simulink model "automata_learning"  (R2022a)
settings: Solver=FixedStepAuto  StartTime=0.0  StopTime=10.0  FixedStep=0.005  RelTol=1e-3
settings Model: Creator=diego  LastModifiedBy=diego

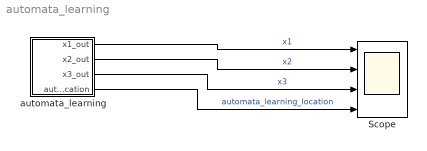
== system automata_learning ==
  Scope : Scope  NumInputPorts=4
  automata_learning : Stateflow chart  TreatAsAtomicUnit=on
  wires:
  automata_learning/1(x1_out) -> Scope/1  "x1"
  automata_learning/2(x2_out) -> Scope/2  "x2"
  automata_learning/3(x3_out) -> Scope/3  "x3"
  automata_learning/4(automata_learning_location) -> Scope/4  "automata_learning_location"

== stateflow chart automata_learning/automata_learning ==
  settings: updateMethod=CONTINUOUS
  state loc1
    du:
    x1_dot = 1801508832791591.0 * x1 * x2 / 9007199254740992.0 - 8444245416915159.0 * x2 / 1125899906842624.0 - 6192709348131975.0 * x3 / 1180591620717411300000.0 - 153051922812249.0 * x1 / 17592186044416.0 + 7205043310630491.0 * x1 * x3 / 72057594037927936.0 + 3602602518173647.0 * x2 * x3 / 36028797018963968.0 + 86143253036817.0 * x1 ^ 2.0 / 18446744073709552000.0 + 6969133893356397.0 * x2 ^ 2.0 / 2361183241434822600000.0 + 2251823042351835.0 * x3 ^ 2.0 / 4503599627370496.0 + 2.7000004841018326;
    x2_dot = 3377693611113005.0 * x1 / 562949953421312.0 + 9007177226223773.0 * x2 / 2251799813685248.0 + 2251818824568175.0 * x3 / 2251799813685248.0 - 7128027310724375.0 * x1 * x2 / 1180591620717411300000.0 + 4052818739806239.0 * x1 * x3 / 590295810358705650000.0 + 1751905182806505.0 * x2 * x3 / 295147905179352830000.0 - 2157835314307409.0 * x1 ^ 2.0 / 590295810358705650000.0 - 3011538389573799.0 * x2 ^ 2.0 / 1180591620717411300000.0 - 7412105066450851.0 * x3 ^ 2.0 / 2361183241434822600000.0 - 5.000004160942135;
    x3_dot = 3377702717258151.0 * x1 / 1125899906842624.0 + 281475456573279.0 * x2 / 140737488355328.0 - 5629502493887539.0 * x3 / 2251799813685248.0 - 2014654941099123.0 * x1 * x2 / 9444732965739290000000.0 + 95050307921055.0 * x1 * x3 / 73786976294838210000.0 + 814066963675827.0 * x2 * x3 / 1180591620717411300000.0 + 2375714488249389.0 * x1 ^ 2.0 / 604462909807314600000000.0 - 7187744990195417.0 * x2 ^ 2.0 / 302231454903657300000000.0 - 5745083834617113.0 * x3 ^ 2.0 / 4722366482869645000000.0 + 0.5000020750789942;
    x1_out=x1;
    x2_out=x2;
    x3_out=x3;
    automata_learning_location =1;
  state loc2
    du:
    x1_dot = 4953956816672575.0 * x1 / 2251799813685248.0 + 4053239121286171.0 * x2 / 1125899906842624.0 + 4391008588697005.0 * x3 / 1125899906842624.0 + 2319261730712697.0 * x1 * x2 / 590295810358705650000.0 + 332132162117049.0 * x1 * x3 / 73786976294838210000.0 + 2383667190927081.0 * x2 * x3 / 295147905179352830000.0 + 3237644951957777.0 * x1 ^ 2.0 / 2361183241434822600000.0 + 4509918697861481.0 * x2 ^ 2.0 / 1180591620717411300000.0 + 5099843972416817.0 * x3 ^ 2.0 / 1180591620717411300000.0 - 0.000000009931971027340576;
    x2_dot = 6755405464511411.0 * x1 / 2251799813685248.0 + 5404321799674583.0 * x2 / 2251799813685248.0 + 7656123947031389.0 * x3 / 2251799813685248.0 - 260928735522237.0 * x1 * x2 / 18446744073709552000.0 - 2240232573594131.0 * x1 * x3 / 147573952589676410000.0 - 7265261209259773.0 * x2 * x3 / 295147905179352830000.0 - 2883771218371389.0 * x1 ^ 2.0 / 288230376151711740.0 - 444013207232747.0 * x2 ^ 2.0 / 36893488147419103000.0 - 7518581652049565.0 * x3 ^ 2.0 / 590295810358705650000.0 + 0.00000004233285259660198;
    x3_dot = 2422790948840695.0 * x1 * x2 / 147573952589676410000.0 - 3039930205138821.0 * x2 / 562949953421312.0 - 3771765751542379.0 * x3 / 562949953421312.0 - 5629502534969053.0 * x1 / 1125899906842624.0 + 5157324152461255.0 * x1 * x3 / 295147905179352830000.0 + 4172107979615031.0 * x2 * x3 / 147573952589676410000.0 + 3445537526208585.0 * x1 ^ 2.0 / 590295810358705650000.0 + 2048261794112287.0 * x2 ^ 2.0 / 147573952589676410000.0 + 2151739806583797.0 * x3 ^ 2.0 / 147573952589676410000.0 - 0.00000004388430930705941;
    x1_out=x1;
    x2_out=x2;
    x3_out=x3;
    automata_learning_location =2;
  loc1 -> loc2 : [3.613 * x1 + 3.088 * x2 - 2.026 * x3 + 1.0 > 0.0]
  (default) -> loc1 : {x1 = 2.5;
      | x2 = -2.5;
      | x3 = 1.2;}
  data: x1_out output; x1 local; x2_out output; x2 local; x3_out output; x3 local; automata_learning_location output
  data x1 settings: updateMethod=SF_CONTINUOUS_TIME_DATA
  data x2 settings: updateMethod=SF_CONTINUOUS_TIME_DATA
  data x3 settings: updateMethod=SF_CONTINUOUS_TIME_DATA
